simulink model "elec_switching_power_supply"  (R2015b)
settings: Solver=ode23t  StartTime=0.0  StopTime=0.006  RelTol=1e-3
PostLoadFcn:
  | controller_choice=1; % Variant selection variable
InitFcn:
  | if ~exist('T_junction1','var')
  |   T_junction1 = 404.79;
  | end
  | if ~exist('T_junction2','var')
  |   T_junction2 = 384.83;
  | end
libraries: fl_lib x14, elec_lib x7, nesl_utility x5
CloseFcn:
  | try close(h1_elec_switching_power_supply), end
  | try close(h2_elec_switching_power_supply), end
  | try clear elec_sps_log tout controller_choice, end
Description:
  | Synchronous Buck Converter
  | 
  | This example shows how to model a switching power supply that converts a 30V DC
  | supply into a regulated 15V DC supply. The model can be used to both size the
  | inductance L and smoothing capacitor C, as well as to design the feedback
  | controller. By selecting between continuous, discrete and fixed-point controllers, the
  | impact of discretization and using limited numerical precision can be explored.
  | 
  | Modeling the switching devices as MOSFETs rather than ideal switches ensures that
  | device on-resistances are correctly represented. The model also captures the
  | switch-on/switch-off timing of the devices, this depending primarily on the gate
  | capacitance values and the PWM driver output resistance.
  | 
  | If you have SimPowerSystems(TM), see example model
  | power_switching_power_supply for an abstracted version of this model that
  | uses ideal switching to give faster simulation times. The model here can be used to
  | determine the on-resistance values required for the ideal switches, plus timing
  | offsets if necessary. Using the ideal switching approach of SimPowerSystems(TM) can
  | be used to simulate more complex power converters.
  | 
  | Workspace variables T_junction1 and T_junction2 are used to define the
  | temperatures at which the two MOSFETs are simulated. Companion models
  | elec_switching_power_supply_thermal and
  | elec_switching_power_supply_thermal_only are used to determine these
  | temperatures.
  | 
  | 
  | 
  | 
  | 
  | 
  | Copyright 2008-2015 The MathWorks, Inc.
settings Model: FPTRunName=Active  Creator=MathWorks  LastModifiedBy=geral
settings DataIOCC: LimitDataPoints=off  SaveFormat=Array  SignalLoggingSaveFormat=ModelDataLogs  SaveOutput=off  SignalLogging=off  DSMLogging=off  SignalLoggingName=sigsOut
settings OptimizationCC: BooleanDataType=off  ExpressionDepthLimit=2147483647  InitFltsAndDblsToZero=on  OptimizeModelRefInitCode=on  LifeSpan=1
settings DebuggingCC: SaveWithParameterizedLinksMsg=none  UnderspecifiedInitializationDetection=Classic  MergeDetectMultiDrivingBlocksExec=none  SignalResolutionControl=TryResolveAllWithWarning  MultiTaskDSMMsg=warning  MultiTaskCondExecSysMsg=none  IntegerOverflowMsg=none  ParameterPrecisionLossMsg=none  FcnCallInpInsideContextMsg=UseLocalSettings  StateNameClashWarn=warning  IntegerSaturationMsg=none
settings HardwareCC: ProdBitPerPointer=32  ProdLargestAtomicFloat=None  ProdIntDivRoundTo=Undefined  ProdEndianess=Unspecified  ProdWordSize=32  ProdHWDeviceType=32-bit Generic
settings RTWCC: SystemTargetFile=ert.tlc  TemplateMakefile=ert_default_tmf  Description=Real-Time Workshop Embedded Coder (no auto configuration)  GenerateReport=on  IncludeHyperlinkInReport=on  LaunchReport=on  CreateSILPILBlock=SIL
settings CodeAppCC: IgnoreCustomStorageClasses=off  CustomSymbolStrType=$N$R$M  InternalIdentifier=Classic
settings ERTTargetCC: TargetFcnLib=ansi_tfl_tmw.mat  GenerateSampleERTMain=on  ERTCustomFileTemplate=example_file_process.tlc
settings ConfigComp: CovModelRefEnable=Off  CovSFcnEnable=off
settings SimscapeCC: SimscapeLogType=all  SimscapeLogName=elec_sps_log  SimscapeLogLimitData=off  SimscapeLogDataHistory=50000

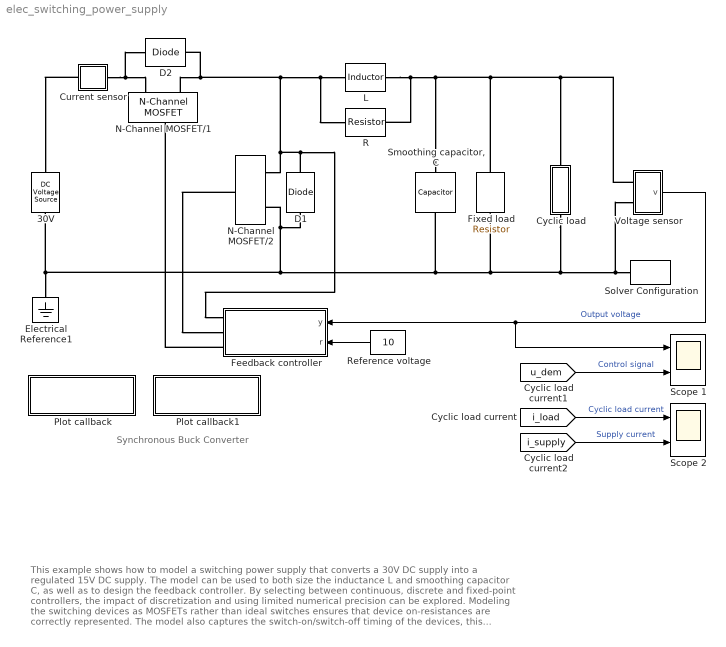
== system elec_switching_power_supply ==
  note: Synchronous Buck Converter
  note: This example shows how to model a switching power supply that converts a 30V DC supply into
      | a regulated 15V DC supply. The model can be used to both size the inductance L and smoothing
      | capacitor C, as well as to design the feedback controller. By selecting between continuous,
      | discrete and fixed-point controllers, the impact of discretization and using limited numerical
      | precision can be explored. Modeling the switching devices as MOSFETs rather than ideal switches
      | ensures that device on-resistances are correctly represented. The model also captures the
      | switch-on/switch-off timing of the devices, this depending primarily on the gate capacitance
      | values and the PWM driver output resistance.
      |
      | If you have SimPowerSystems(TM), see example model power_switching_power_supply for an
      | abstracted version of this model that uses ideal switching to give faster simulation times. The
      | model here can be used to determine the on-resistance values required for the ideal switches,
      | plus timing offsets if necessary. Using the ideal switching approach of SimPowerSystems can be
      | used to simulate more complex power converters.
      |
      | Workspace variables T_junction1 and T_junction2 are used to define the temperatures at which
      | the two MOSFETs are simulated. Companion models elec_switching_power_supply_thermal
      | and elec_switching_power_supply_thermal_only are used to determine these temperatures.
  30V : fl_lib/Electrical/Electrical Sources/DC Voltage Source  v0=18 V
  Current sensor : Subsystem
  Cyclic load : Subsystem
  D1 : elec_lib/Semiconductor Devices/Diode  ModelType=3  Vf=0.6 V  Ron=0.3 Ohm  Goff=1e-8 S  Rz=0.3 Ohm  Vz=50 V  C_PWL=5 pF  prmExp=1  I12=[ 0.25 5 ] A  V12=[ 0.7 0.8 ] V  I1=0.07 A  V1=0.7 V  RS=0.01 Ohm  IS=1e-14 A  Tmeas=25 C  ec=1  BV=Inf V  C_param=1  CJ0=100 pF  VJ=1 V  Mgrad=0.5  Vvec=[ 0.1 10 100 ] V  Cvec=[ 3.5 1 0.4 ] pF  FC=0.5  Q_param=1  Irrm=-7.15 A  iF=4 A  didt=-750 A/us  trr=115 ns  TT=50 ns  tau=100 ns  T_param=1  IS_T2=1.25e-7 A  I1_T2=0.245 A  V1_T2=0.5 V  Tmeas2=125 C  EG_param=1  EG=1.11 eV  XTI_param=1  XTI=3  dBVdT=0 V/K  Tdevice=25 C  Rth=[ 0 10 ] K/W  thermal_mass_parameterization=1  thermal_mass=[ 0 1 ] J/K  thermal_time_constant=[ 0 10 ] s  thermal_mass_initial_temperatures=[ 25 25 ] C
  D2 : elec_lib/Semiconductor Devices/Diode  ModelType=3  Vf=0.6 V  Ron=0.3 Ohm  Goff=1e-8 S  Rz=0.3 Ohm  Vz=50 V  C_PWL=5 pF  prmExp=1  I12=[ 0.25 5 ] A  V12=[ 0.7 0.8 ] V  I1=0.07 A  V1=0.7 V  RS=0.01 Ohm  IS=1e-14 A  Tmeas=25 C  ec=1  BV=Inf V  C_param=1  CJ0=100 pF  VJ=1 V  Mgrad=0.5  Vvec=[ 0.1 10 100 ] V  Cvec=[ 3.5 1 0.4 ] pF  FC=0.5  Q_param=1  Irrm=-7.15 A  iF=4 A  didt=-750 A/us  trr=115 ns  TT=50 ns  tau=100 ns  T_param=1  IS_T2=1.25e-7 A  I1_T2=0.245 A  V1_T2=0.5 V  Tmeas2=125 C  EG_param=1  EG=1.11 eV  XTI_param=1  XTI=3  dBVdT=0 V/K  Tdevice=25 C  Rth=[ 0 10 ] K/W  thermal_mass_parameterization=1  thermal_mass=[ 0 1 ] J/K  thermal_time_constant=[ 0 10 ] s  thermal_mass_initial_temperatures=[ 25 25 ] C
  Electrical Reference1 : fl_lib/Electrical/Electrical Elements/Electrical Reference
  Feedback controller : Subsystem
  Fixed load : fl_lib/Electrical/Electrical Elements/Resistor  R=2.4 Ohm  i_specify=off  i_priority=High  i=0 A  v_specify=off  v_priority=High  v=0 V
  L : fl_lib/Electrical/Electrical Elements/Inductor  l=22e-6 H  r=0 Ohm  g=0 1/Ohm  i_specify=off  i_priority=High  i=0 A  v_specify=off  v_priority=High  v=0 V  i_L_specify=on  i_L_priority=High  i_L=0 A
  N-Channel MOSFET/1 : elec_lib/Semiconductor Devices/N-Channel MOSFET  parameterization=1  prmDatasheet=2  prmEquCoeff=1  Beta=5 A/V^2  Rds=0.1 Ohm  Id=6 A  Vgs=15 V  Vth=2 V  lam=0 1/V  Tmeas=25 C  RS=0.01 Ohm  RD=0.01 Ohm  C_param=1  C_GS=270 pF  C_GD=80 pF  C_iss=350 pF  C_rss=80 pF  C_oss=0 pF  C_GS_vec=[ 270 300 290 280 295 255 ] pF  C_GD_vec=[ 450 400 300 190 95 55 ] pF  C_iss_vec=[ 720 700 590 470 390 310 ] pF  C_rss_vec=[ 450 400 300 190 95 55 ] pF  C_oss_vec=[ 900 810 690 420 270 170 ] pF  C_Vds_vec=[ 0.1 0.3 1 3 10 30 ] V  charge_linearity_param=1  C_OX=200 pF  V_C_OX=-0.5 V  dVth_dT=-6 mV/K  Rds_T2=0.2 Ohm  Tmeas2=125 C  BEXDatasheet=-1.5  BEXEquCoeff=-1.5  TdeviceDatasheet=T_junction1 K  TdeviceEquCoeff=25 C  Rth=[ 20 1 ] K/W  thermal_mass_parameterization=2  thermal_mass=[ 0.3 2 ] J/K  thermal_time_constant=[ 1 10 ] s  thermal_mass_initial_temperatures=[ 300 300 ] K
  N-Channel MOSFET/2 : elec_lib/Semiconductor Devices/N-Channel MOSFET  parameterization=1  prmDatasheet=2  prmEquCoeff=1  Beta=5 A/V^2  Rds=0.1 Ohm  Id=6 A  Vgs=15 V  Vth=2 V  lam=0 1/V  Tmeas=25 C  RS=0.01 Ohm  RD=0.01 Ohm  C_param=1  C_GS=270 pF  C_GD=80 pF  C_iss=350 pF  C_rss=80 pF  C_oss=0 pF  C_GS_vec=[ 270 300 290 280 295 255 ] pF  C_GD_vec=[ 450 400 300 190 95 55 ] pF  C_iss_vec=[ 720 700 590 470 390 310 ] pF  C_rss_vec=[ 450 400 300 190 95 55 ] pF  C_oss_vec=[ 900 810 690 420 270 170 ] pF  C_Vds_vec=[ 0.1 0.3 1 3 10 30 ] V  charge_linearity_param=1  C_OX=200 pF  V_C_OX=-0.5 V  dVth_dT=-6 mV/K  Rds_T2=0.2 Ohm  Tmeas2=125 C  BEXDatasheet=-1.5  BEXEquCoeff=-1.5  TdeviceDatasheet=T_junction2 K  TdeviceEquCoeff=25 C  Rth=[ 20 1 ] K/W  thermal_mass_parameterization=2  thermal_mass=[ 0.3 2 ] J/K  thermal_time_constant=[ 1 10 ] s  thermal_mass_initial_temperatures=[ 300 300 ] K
  Plot callback : Subsystem
      settings: OpenFcn=|
      | if exist('elec_sps_log','var')
      |     elec_switching_power_supply_plots
      | else
      |     disp('Run the model first to generate results')
      | end
      mask Display: disp('Plot logged data')
  Plot callback1 : Subsystem
      settings: OpenFcn=open('elec_switching_power_supply_plots.m')
      mask Display: disp('Open plot file')
  R : fl_lib/Electrical/Electrical Elements/Resistor  R=10 kOhm  i_specify=off  i_priority=High  i=0 A  v_specify=off  v_priority=High  v=0 V
  Reference voltage : Constant  Value=10
  Scope 1 : Scope  NumInputPorts=2
  Scope 2 : Scope  NumInputPorts=2
  "Smoothing capacitor, C" : fl_lib/Electrical/Electrical Elements/Capacitor  c=220 uF  r=0 Ohm  g=0 1/Ohm  i_specify=off  i_priority=High  i=0 A  v_specify=off  v_priority=High  v=0 V  vc_specify=on  vc_priority=High  vc=0 V
  Solver Configuration : nesl_utility/Solver Configuration  PhysicalDomain=network_engine_domain  SubClassName=solver  LeftPortType=input  RightPortType=generic  Accelerate=off  Tones=[]  Harmonics=[]  SimulateNoise=off  Profile=off  UseLocalSampling=off  EnableSwitchedLinearOptims=on  FrequencyDomain=off  UseCCode=off  RelTol=0.001  AbsTol=1e-06  MinStep=1e-09  ToWorkspace=off  RevertToSquareIcSolve=off  NumHomotopyIterations=100  PhasorMode=off  PhasorModeNumHarmonics=1  DoDC=off  ResidualTolerance=1e-9  UseLocalSolver=off  LocalSolverChoice=NE_BACKWARD_EULER_ADVANCER  LocalSolverSampleTime=1e-7  DoFixedCost=off  MaxNonlinIter=12  MaxModeIter=2  LinearAlgebra=Sparse  DelaysMemoryBudget=1024  AutomaticFiltering=on  FilteringTimeConstant=0.001
  Voltage sensor : Subsystem
      settings: CopyFcn=set_param(gcb,'LinkStatus','none')
  wires:
  Reference voltage/1 -> Feedback controller/2(r)
  Voltage sensor/1(v) -> Feedback controller/1(y), Scope 1/1  "Output voltage"
  [u_dem] -> Scope 1/2  "Control signal"
  [i_load] -> Scope 2/1  "Cyclic load current"
  [i_supply] -> Scope 2/2  "Supply current"
  connections:
  N-Channel MOSFET/1/RConn2 -- L/RConn1 -- R/RConn1 -- D1/RConn1 -- Feedback controller/RConn1 -- N-Channel MOSFET/2/RConn1 -- D2/LConn1
  Voltage sensor/LConn1 -- "Smoothing capacitor, C"/LConn1 -- R/LConn1 -- L/LConn1 -- Fixed load/LConn1 -- Cyclic load/RConn1
  N-Channel MOSFET/2/RConn2 -- D1/LConn1 -- Cyclic load/LConn1 -- Voltage sensor/LConn2 -- Solver Configuration/RConn1 -- Fixed load/RConn1 -- "Smoothing capacitor, C"/RConn1 -- 30V/RConn1 -- Electrical Reference1/LConn1
  Feedback controller/RConn3 -- N-Channel MOSFET/1/LConn1
  N-Channel MOSFET/2/LConn1 -- Feedback controller/RConn2
  Current sensor/LConn1 -- 30V/LConn1
  Current sensor/RConn1 -- N-Channel MOSFET/1/RConn1 -- D2/RConn1

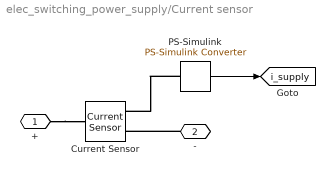
== system elec_switching_power_supply/Current sensor ==
  Current Sensor : fl_lib/Electrical/Electrical Sensors/Current Sensor
  PS-Simulink : nesl_utility/PS-Simulink Converter  PhysicalDomain=network_engine_domain  SubClassName=ps_output  LeftPortType=input  RightPortType=output  PseudoPeriodic=off  Frequencies=[]  Unit=A  AffineConversion=off
  + : PMIOPort  Port=1  Side=Left
  - : PMIOPort  Port=2  Side=Right
  tag scope: i_supply=global
  wires:
  PS-Simulink/1 -> [i_supply]
  connections:
  PS-Simulink/LConn1 -- Current Sensor/RConn1
  +/RConn1 -- Current Sensor/LConn1
  -/RConn1 -- Current Sensor/RConn2

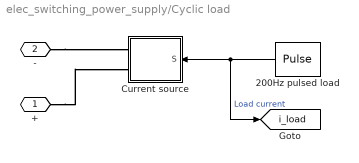
== system elec_switching_power_supply/Cyclic load ==
  200Hz pulsed load : DiscretePulseGenerator  PulseType=Time based  Period=1/200  PulseWidth=50  PhaseDelay=1/400
  Current source : Subsystem
      settings: CopyFcn=set_param(gcb,'LinkStatus','none')
  + : PMIOPort  Port=1  Side=Right
  - : PMIOPort  Port=2  Side=Left
  tag scope: i_load=global
  wires:
  200Hz pulsed load/1 -> [i_load], Current source/1(S)  "Load current"
  connections:
  +/RConn1 -- Current source/RConn2
  -/RConn1 -- Current source/RConn1

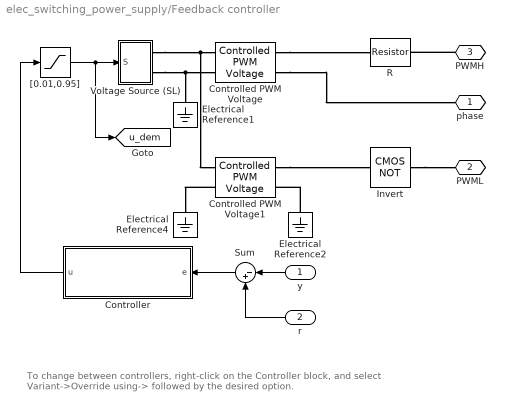
== system elec_switching_power_supply/Feedback controller ==
  note: To change between controllers, right-click on the Controller block,
      | and select Variant->Override using-> followed by the desired option.
  y : Inport
  r : Inport  Port=2
  Controlled PWM Voltage : elec_lib/Actuators & Drivers/Drivers/Controlled PWM Voltage  F=100 kHz  TD=0 s  pulse_width_offset=0 s  Vmin=0 V  Vmax=1 V  Vm=30 V  pwm_or_av=1  event_type=1  sample_time=1e-6 s
  Controlled PWM Voltage1 : elec_lib/Actuators & Drivers/Drivers/Controlled PWM Voltage  F=50 kHz  TD=0 s  pulse_width_offset=0 s  Vmin=0 V  Vmax=1 V  Vm=30 V  pwm_or_av=1  event_type=1  sample_time=1e-6 s
  Controller : Subsystem  Variant=on  OverrideUsingVariant=controller_choice==3
      settings: AttributesFormatString=%<BlockChoice>
  Electrical Reference1 : fl_lib/Electrical/Electrical Elements/Electrical Reference
  Electrical Reference2 : fl_lib/Electrical/Electrical Elements/Electrical Reference
  Electrical Reference4 : fl_lib/Electrical/Electrical Elements/Electrical Reference
  Invert : elec_lib/Integrated Circuits/Logic/CMOS NOT  V_IL=10 V  V_IH=20 V  C_IN=0 pF  output_type=1  V_OL=0 V  V_OH=30 V  V_CC=5 V  V_meas=5 V  R_OUT=100 Ohm  R_OH=[ 25 250 ] Ohm  I_OH=63 mA  R_OL=[ 30 800 ] Ohm  I_OL=-45 mA  Delay=0 s  Ron=5 Ohm  Vf=0.6 V  output_state=1
  R : fl_lib/Electrical/Electrical Elements/Resistor  R=100 Ohm  i_specify=off  i_priority=High  i=0 A  v_specify=off  v_priority=High  v=0 V
  Sum : Sum  Inputs=|-+  SaturateOnIntegerOverflow=on  InputSameDT=on  OutDataTypeStr=Inherit: Same as first input
  Voltage Source (SL) : Subsystem
      settings: CopyFcn=set_param(gcb,'LinkStatus','none')
  "[0.01,0.95]" : Saturate  UpperLimit=0.95  LowerLimit=.01
  phase : PMIOPort  Port=1  Side=Right
  PWML : PMIOPort  Port=2  Side=Right
  PWMH : PMIOPort  Port=3  Side=Right
  tag scope: u_dem=global
  wires:
  r/1 -> Sum/2
  y/1 -> Sum/1
  Sum/1 -> Controller/1(e)
  "[0.01,0.95]"/1 -> Voltage Source (SL)/1(S), [u_dem]
  Controller/1(u) -> "[0.01,0.95]"/1
  connections:
  Voltage Source (SL)/RConn1 -- Controlled PWM Voltage1/LConn1 -- Controlled PWM Voltage/LConn1
  Voltage Source (SL)/RConn2 -- Controlled PWM Voltage/LConn2 -- Electrical Reference1/LConn1
  Controlled PWM Voltage/RConn2 -- phase/RConn1
  Controlled PWM Voltage/RConn1 -- R/RConn1
  PWMH/RConn1 -- R/LConn1
  Invert/RConn1 -- PWML/RConn1
  Controlled PWM Voltage1/RConn1 -- Invert/LConn1
  Electrical Reference2/LConn1 -- Controlled PWM Voltage1/RConn2
  Controlled PWM Voltage1/LConn2 -- Electrical Reference4/LConn1

== system elec_switching_power_supply/Plot callback ==

== system elec_switching_power_supply/Plot callback1 ==

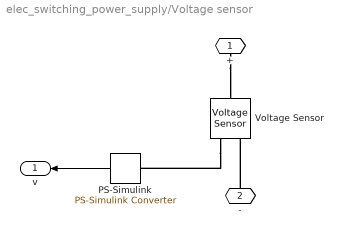
== system elec_switching_power_supply/Voltage sensor ==
  PS-Simulink : nesl_utility/PS-Simulink Converter  PhysicalDomain=network_engine_domain  SubClassName=ps_output  LeftPortType=input  RightPortType=output  PseudoPeriodic=off  Frequencies=[]  Unit=V  AffineConversion=off
  Voltage Sensor : fl_lib/Electrical/Electrical Sensors/Voltage Sensor
  + : PMIOPort  Port=1  Side=Left
  - : PMIOPort  Port=2  Side=Left
  v : Outport
  wires:
  PS-Simulink/1 -> v/1
  connections:
  Voltage Sensor/RConn1 -- PS-Simulink/LConn1
  +/RConn1 -- Voltage Sensor/LConn1
  -/RConn1 -- Voltage Sensor/RConn2

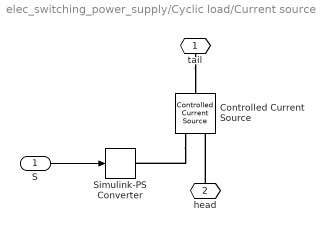
== system elec_switching_power_supply/Cyclic load/Current source ==
  S : Inport
  Controlled Current Source : fl_lib/Electrical/Electrical Sources/Controlled Current Source
  Simulink-PS Converter : nesl_utility/Simulink-PS Converter  PhysicalDomain=network_engine_domain  SubClassName=ps_input  LeftPortType=input  RightPortType=output  PseudoPeriodic=off  Frequencies=[]  NoiseDistribution=none  NoiseParameters=[]  Unit=A  AffineConversion=off  InputFiltering=off  SimscapeFilterOrder=1  InputFilterTimeConstant=.001  UdotUserProvided=0
  tail : PMIOPort  Port=1  Side=Right
  head : PMIOPort  Port=2  Side=Right
  wires:
  S/1 -> Simulink-PS Converter/1
  connections:
  tail/RConn1 -- Controlled Current Source/LConn1
  head/RConn1 -- Controlled Current Source/RConn2
  Controlled Current Source/RConn1 -- Simulink-PS Converter/RConn1

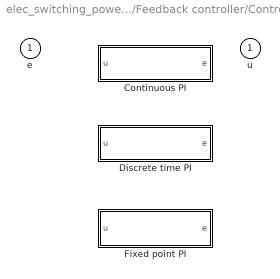
== system elec_switching_power_supply/Feedback controller/Controller ==
  e : Inport
  Continuous PI : Subsystem  VariantControl=controller_choice==1
  Discrete time PI : Subsystem  VariantControl=controller_choice==2
  Fixed point PI : Subsystem  MinMaxOverflowLogging=MinMaxAndOverflow  VariantControl=controller_choice==3
  u : Outport

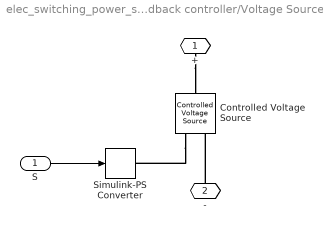
== system elec_switching_power_supply/Feedback controller/Voltage Source (SL) ==
  S : Inport
  Controlled Voltage Source : fl_lib/Electrical/Electrical Sources/Controlled Voltage Source
  Simulink-PS Converter : nesl_utility/Simulink-PS Converter  PhysicalDomain=network_engine_domain  SubClassName=ps_input  LeftPortType=input  RightPortType=output  PseudoPeriodic=off  Frequencies=[]  NoiseDistribution=none  NoiseParameters=[]  Unit=V  AffineConversion=off  InputFiltering=off  SimscapeFilterOrder=1  InputFilterTimeConstant=.001  UdotUserProvided=0
  + : PMIOPort  Port=1  Side=Right
  - : PMIOPort  Port=2  Side=Right
  wires:
  S/1 -> Simulink-PS Converter/1
  connections:
  +/RConn1 -- Controlled Voltage Source/LConn1
  -/RConn1 -- Controlled Voltage Source/RConn2
  Controlled Voltage Source/RConn1 -- Simulink-PS Converter/RConn1

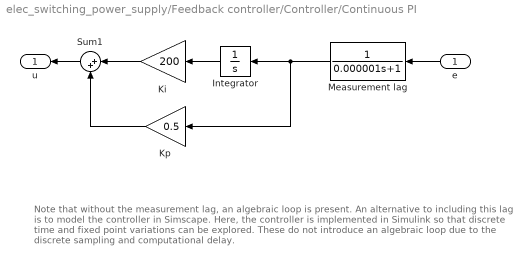
== system elec_switching_power_supply/Feedback controller/Controller/Continuous PI ==
  note: Note that without the measurement lag, an algebraic loop is present. An alternative to
      | including this lag is to model the controller in Simscape. Here, the controller is implemented
      | in Simulink so that discrete time and fixed point variations can be explored. These do not
      | introduce an algebraic loop due to the discrete sampling and computational delay.
  e : Inport
  Integrator : Integrator
  Ki : Gain  Gain=200
  Kp : Gain  Gain=0.5
  Measurement lag : TransferFcn  Denominator=[0.000001 1]
  Sum1 : Sum  Inputs=|++  SaturateOnIntegerOverflow=on  InputSameDT=on  OutDataTypeStr=Inherit: Same as first input
  u : Outport
  wires:
  Measurement lag/1 -> Integrator/1, Kp/1
  Ki/1 -> Sum1/1
  Sum1/1 -> u/1
  Kp/1 -> Sum1/2
  Integrator/1 -> Ki/1
  e/1 -> Measurement lag/1

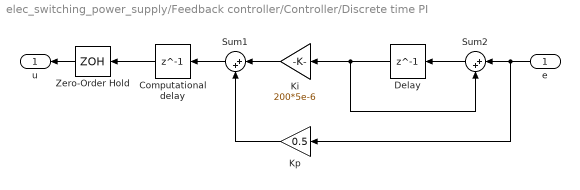
== system elec_switching_power_supply/Feedback controller/Controller/Discrete time PI ==
  e : Inport
  Computational delay : Delay  DelayLength=1  InputProcessing=Inherited  SampleTime=5e-6
  Delay : Delay  DelayLength=1  InputProcessing=Inherited  SampleTime=5e-6
  Ki : Gain  Gain=200*5e-6
  Kp : Gain  Gain=0.5
  Sum1 : Sum  Inputs=|++  SaturateOnIntegerOverflow=on  InputSameDT=on  OutDataTypeStr=Inherit: Same as first input
  Sum2 : Sum  Inputs=|++  SaturateOnIntegerOverflow=on  InputSameDT=on  OutDataTypeStr=Inherit: Same as first input
  Zero-Order Hold : ZeroOrderHold  SampleTime=5e-6
  u : Outport
  wires:
  Ki/1 -> Sum1/1
  Sum2/1 -> Delay/1
  Delay/1 -> Ki/1, Sum2/2
  Kp/1 -> Sum1/2
  Sum1/1 -> Computational delay/1
  e/1 -> Sum2/1, Kp/1
  Zero-Order Hold/1 -> u/1
  Computational delay/1 -> Zero-Order Hold/1

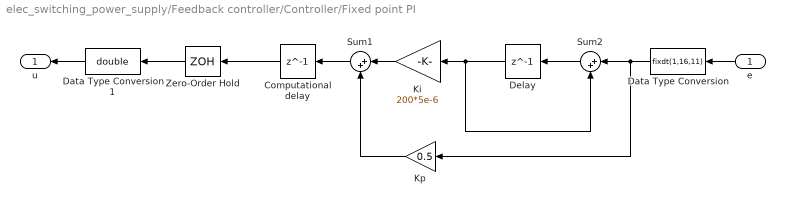
== system elec_switching_power_supply/Feedback controller/Controller/Fixed point PI ==
  e : Inport
  Computational delay : Delay  DelayLength=1  InputProcessing=Inherited  SampleTime=50e-6
  Data Type Conversion : DataTypeConversion  OutDataTypeStr=fixdt(1,16,11)  RndMeth=Nearest
  Data Type Conversion1 : DataTypeConversion  OutDataTypeStr=double  RndMeth=Nearest
  Delay : Delay  DelayLength=1  InputProcessing=Inherited  SampleTime=50e-6
  Ki : Gain  Gain=200*5e-6  OutDataTypeStr=fixdt(1,16,13)  RndMeth=Nearest
  Kp : Gain  Gain=0.5  OutDataTypeStr=fixdt(1,16,9)  RndMeth=Nearest
  Sum1 : Sum  Inputs=|++  SaturateOnIntegerOverflow=on
  Sum2 : Sum  Inputs=|++  SaturateOnIntegerOverflow=on  InputSameDT=on  OutDataTypeStr=Inherit: Same as first input
  Zero-Order Hold : ZeroOrderHold  SampleTime=50e-6
  u : Outport
  wires:
  Ki/1 -> Sum1/1
  Data Type Conversion1/1 -> u/1
  Data Type Conversion/1 -> Sum2/1, Kp/1
  Sum1/1 -> Computational delay/1
  Kp/1 -> Sum1/2
  e/1 -> Data Type Conversion/1
  Delay/1 -> Ki/1, Sum2/2
  Sum2/1 -> Delay/1
  Computational delay/1 -> Zero-Order Hold/1
  Zero-Order Hold/1 -> Data Type Conversion1/1
